simulink model "Practica2"  (R2024b)
settings: Solver=VariableStepAuto  StartTime=0.0  StopTime=20.0  RelTol=1e-3
InitFcn:
  | Ip = 0.0079;
  | Mc = 0.7031;
  | lp = 0.3302;
  | Mp = 0.23;
  | Fc = 0;
  | Beq = 4.3;
  | G = 9.81;
  | Bp = 0.0024;
  | A = deg2rad(1);
  | Xc = 0;
  | dA = 0;
  | dXc = 0;
settings Model: Creator=RAM  LastModifiedBy=RAM

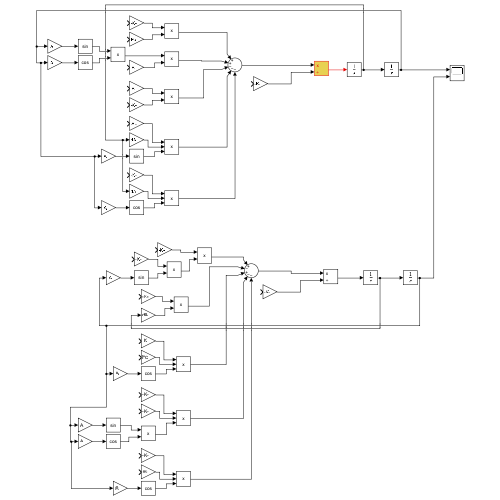
[thumbnail: Simulink's stored preview of the top-level diagram]
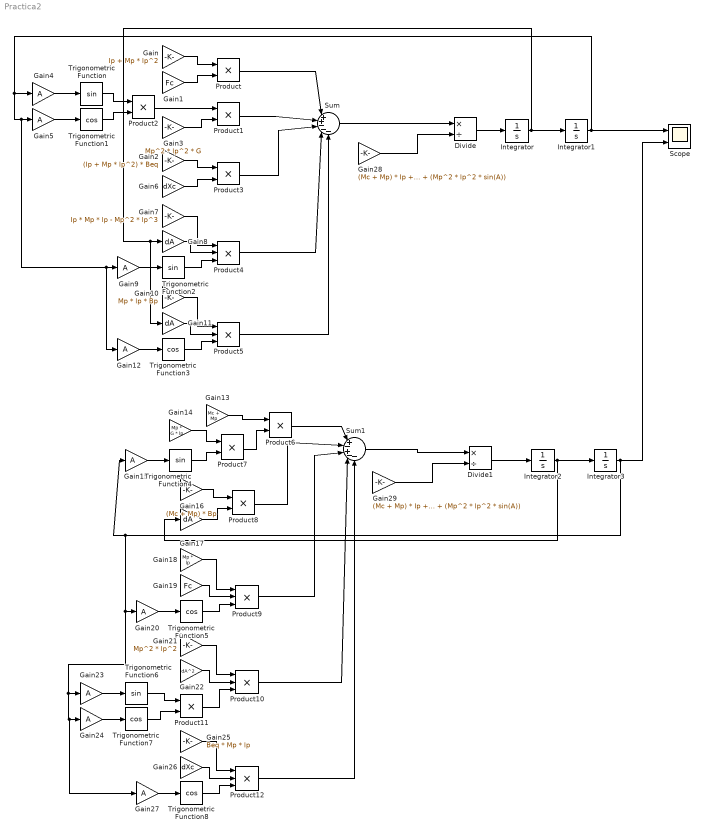
== system Practica2 ==
  Divide : Product  Inputs=*/
  Divide1 : Product  Inputs=*/
  Gain : Gain  Gain=Ip + Mp * lp^2
  Gain1 : Gain  Gain=Fc
  Gain10 : Gain  Gain=Mp * lp * Bp
  Gain11 : Gain  Gain=dA
  Gain{4..5,9,12,15,20,23..24,27} (9 alike) : Gain  Gain=A
  Gain13 : Gain  Gain=Mc + Mp
  Gain14 : Gain  Gain=Mp * G * lp
  Gain16 : Gain  Gain=(Mc + Mp) * Bp
  Gain17 : Gain  Gain=dA
  Gain18 : Gain  Gain=Mp * lp
  Gain19 : Gain  Gain=Fc
  Gain2 : Gain  Gain=(Ip + Mp * lp^2) * Beq
  Gain21 : Gain  Gain=Mp^2 * lp^2
  Gain22 : Gain  Gain=dA^2
  Gain25 : Gain  Gain=Beq * Mp * lp
  Gain26 : Gain  Gain=dXc
  Gain28 : Gain  Gain=(Mc + Mp) * Ip + (Mc * Mp * lp^2) + (Mp^2 * lp^2 * sin(A))
  Gain29 : Gain  Gain=(Mc + Mp) * Ip + (Mc * Mp * lp^2) + (Mp^2 * lp^2 * sin(A))
  Gain3 : Gain  Gain=Mp^2 * lp^2 * G
  Gain6 : Gain  Gain=dXc
  Gain7 : Gain  Gain=Ip * Mp * lp - Mp^2 * lp^3
  Gain8 : Gain  Gain=dA
  Integrator : Integrator  InitialCondition=dA
  Integrator1 : Integrator  InitialCondition=A
  Integrator2 : Integrator  InitialCondition=dA
  Integrator3 : Integrator  InitialCondition=A
  Product{,1..3,6..8,11} (8 alike) : Product
  Product{4..5,9..10,12} (5 alike) : Product  Inputs=3
  Scope : Scope  NumInputPorts=2
  Sum : Sum  Inputs=|++---
  Sum1 : Sum  Inputs=|+-+--
  Trigonometric Function{,2,4,6} (4 alike) : Trigonometry
  Trigonometric Function{1,3,5,7..8} (5 alike) : Trigonometry  Operator=cos
  wires:
  Gain1/1 -> Product/2
  Gain/1 -> Product/1
  Product/1 -> Sum/1
  Product1/1 -> Sum/2
  Trigonometric Function1/1 -> Product2/2
  Trigonometric Function/1 -> Product2/1
  Gain5/1 -> Trigonometric Function1/1
  Gain4/1 -> Trigonometric Function/1
  Product2/1 -> Product1/1
  Gain3/1 -> Product1/2
  Gain2/1 -> Product3/1
  Gain6/1 -> Product3/2
  Product3/1 -> Sum/3
  Gain8/1 -> Product4/2
  Gain7/1 -> Product4/1
  Gain9/1 -> Trigonometric Function2/1
  Trigonometric Function2/1 -> Product4/3
  Product4/1 -> Sum/4
  Gain10/1 -> Product5/1
  Gain11/1 -> Product5/2
  Trigonometric Function3/1 -> Product5/3
  Gain12/1 -> Trigonometric Function3/1
  Product5/1 -> Sum/5
  Gain15/1 -> Trigonometric Function4/1
  Gain14/1 -> Product7/1
  Trigonometric Function4/1 -> Product7/2
  Product7/1 -> Product6/2
  Gain13/1 -> Product6/1
  Product6/1 -> Sum1/1
  Gain17/1 -> Product8/2
  Gain16/1 -> Product8/1
  Product8/1 -> Sum1/2
  Trigonometric Function5/1 -> Product9/3
  Gain18/1 -> Product9/1
  Gain20/1 -> Trigonometric Function5/1
  Gain19/1 -> Product9/2
  Product9/1 -> Sum1/3
  Gain22/1 -> Product10/2
  Gain21/1 -> Product10/1
  Gain24/1 -> Trigonometric Function7/1
  Trigonometric Function7/1 -> Product11/2
  Trigonometric Function6/1 -> Product11/1
  Gain23/1 -> Trigonometric Function6/1
  Product11/1 -> Product10/3
  Product10/1 -> Sum1/4
  Gain26/1 -> Product12/2
  Gain25/1 -> Product12/1
  Trigonometric Function8/1 -> Product12/3
  Gain27/1 -> Trigonometric Function8/1
  Product12/1 -> Sum1/5
  Sum/1 -> Divide/1
  Gain28/1 -> Divide/2
  Gain29/1 -> Divide1/2
  Sum1/1 -> Divide1/1
  Divide/1 -> Integrator/1
  Integrator/1 -> Integrator1/1, Gain11/1, Gain8/1
  Integrator1/1 -> Gain12/1, Gain9/1, Gain5/1, Gain4/1, Scope/1
  Integrator2/1 -> Gain17/1, Integrator3/1
  Divide1/1 -> Integrator2/1
  Integrator3/1 -> Gain27/1, Gain24/1, Gain23/1, Gain20/1, Gain15/1, Scope/2
